simulink model "SimulinkTest"  (Simulink 7.5)
settings: Solver=FixedStepDiscrete  StartTime=0.0  StopTime=Inf  FixedStep=.01  RelTol=1e-3
libraries: instrumentlib x2, aerolibanimutils x1
settings Model: Creator=Bryant  LastModifiedBy=Bryant

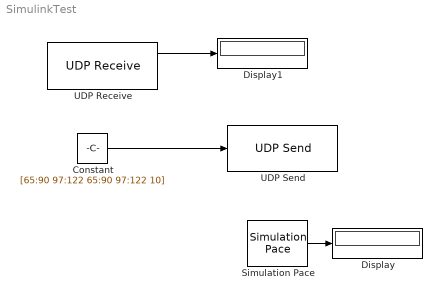
== system SimulinkTest ==
  Constant : Constant  Value=[65:90 97:122 65:90 97:122 10]  OutDataTypeMode=uint8  OutDataType=fixdt(1, 16)  OutScaling=2^0  OutDataTypeStr=uint8  SampleTime=.04
  Display : Display
  Display1 : Display
  Simulation Pace : aerolibanimutils/Simulation Pace  SimulationPace=1  SleepMode=MATLAB Thread  OutputPaceError=on  SampleTime=.01
      settings: AttributesFormatString=%<SimulationPace> sec/sec
  UDP Receive : instrumentlib/UDP Receive  DialogController=instrumentcreatedialog  DialogControllerArgs=DataTag0  Host=127.0.0.1  Port=1301  LocalPort=-1  DataSize=[1 1]  EnableBlockingMode=off  Timeout=10  SampleTime=0.01  DataType=uint8  ByteOrder=BigEndian
  UDP Send : instrumentlib/UDP Send  DialogController=instrumentcreatedialog  DialogControllerArgs=DataTag1  Host=127.0.0.1  Port=1300  LocalPort=-1  EnableBlockingMode=off  ByteOrder=BigEndian
  wires:
  Constant/1 -> UDP Send/1
  Simulation Pace/1 -> Display/1
  UDP Receive/1 -> Display1/1
